simulink library "Surface_Mu_Axle3_LUT_Pos"  (R2026a)
settings: Solver=VariableStepAuto
undefined symbols (not defined in the file or in its folder): Scene
libraries: Tire_Utilities x6
Description:
  | Simscape Vehicle Templates Library
  | 
  | Copyright 2018-2024 The MathWorks, Inc.
settings Model: Creator=smiller  LastModifiedBy=smiller

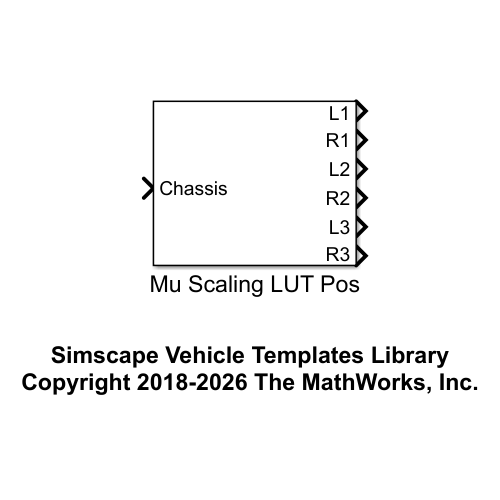
[thumbnail: Simulink's stored preview of the top-level diagram]
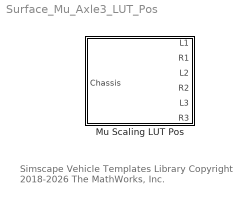
== system Surface_Mu_Axle3_LUT_Pos ==
  note: Simscape Vehicle Templates Library
      | Copyright 2018-2026 The MathWorks, Inc.
  Mu Scaling LUT Pos : Subsystem  VariantControl=Choice  mask(Scale Friction Coefficient by Position){xposL1=Scene.Mu_Scaling.x, yposL1=Scene.Mu_Scaling.y, ScaleTableL1=Scene.Mu_Scaling.scale, xposR1=Scene.Mu_Scaling.x, yposR1=Scene.Mu_Scaling.y, ScaleTableR1=Scene.Mu_Scaling.scale, xposL2=Scene.Mu_Scaling.x, yposL2=Scene.Mu_Scaling.y, ScaleTableL2=Scene.Mu_Scaling.scale, xposR2=Scene.Mu_Scaling.x, yposR2=Scene.Mu_Scaling.y, ScaleTableR2=Scene.Mu_Scaling.scale, xposL3=Scene.Mu_Scaling.x, yposL3=Scene.Mu_Scaling.y, ScaleTableL3=Scene.Mu_Scaling.scale, xposR3=Scene.Mu_Scaling.x, yposR3=Scene.Mu_Scaling.y, ScaleTableR3=Scene.Mu_Scaling.scale}
      mask help: Determines scaling factor for friction coefficient based on wheel x-y position.
      mask TypeOptions xposL1: LUT Scale L1/BreakpointsForDimension1
      mask TypeOptions yposL1: LUT Scale L1/BreakpointsForDimension2
      mask TypeOptions ScaleTableL1: LUT Scale L1/Table
      mask TypeOptions xposR1: LUT Scale R1/BreakpointsForDimension1
      mask TypeOptions yposR1: LUT Scale R1/BreakpointsForDimension2
      mask TypeOptions ScaleTableR1: LUT Scale R1/Table
      mask TypeOptions xposL2: LUT Scale L2/BreakpointsForDimension1
      mask TypeOptions yposL2: LUT Scale L2/BreakpointsForDimension2
      mask TypeOptions ScaleTableL2: LUT Scale L2/Table
      mask TypeOptions xposR2: LUT Scale R2/BreakpointsForDimension1
      mask TypeOptions yposR2: LUT Scale R2/BreakpointsForDimension2
      mask TypeOptions ScaleTableR2: LUT Scale R2/Table
      mask TypeOptions xposL3: LUT Scale L3/BreakpointsForDimension1
      mask TypeOptions yposL3: LUT Scale L3/BreakpointsForDimension2
      mask TypeOptions ScaleTableL3: LUT Scale L3/Table
      mask TypeOptions xposR3: LUT Scale R3/BreakpointsForDimension1
      mask TypeOptions yposR3: LUT Scale R3/BreakpointsForDimension2
      mask TypeOptions ScaleTableR3: LUT Scale R3/Table
      mask DialogControl text_whl Prompt: Wheel
      mask DialogControl text_xpos Prompt: X [1xm] (m)
      mask DialogControl text_ypos Prompt: Y [1xn] (m)
      mask DialogControl text_mu Prompt: Scale [mxn] (m)
      mask DialogControl text_L1 Prompt: L1
      mask DialogControl text_R1 Prompt: R1
      mask DialogControl text_L2 Prompt: L2
      mask DialogControl text_R2 Prompt: R2
      mask DialogControl text_L3 Prompt: L3
      mask DialogControl text_R3 Prompt: R3

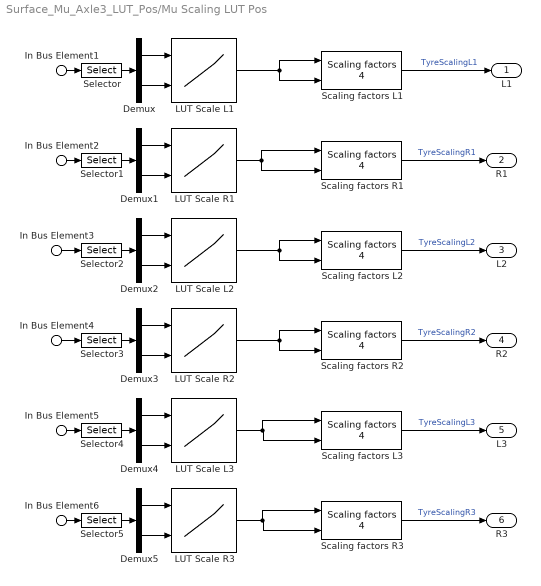
== system Surface_Mu_Axle3_LUT_Pos/Mu Scaling LUT Pos ==
  In Bus Element1 : Inport  PortName=Chassis  Element=WhlL1.xyz
  In Bus Element2 : Inport  PortName=Chassis  Element=WhlR1.xyz
  In Bus Element3 : Inport  PortName=Chassis  Element=WhlL2.xyz
  In Bus Element4 : Inport  PortName=Chassis  Element=WhlR2.xyz
  In Bus Element5 : Inport  PortName=Chassis  Element=WhlL3.xyz
  In Bus Element6 : Inport  PortName=Chassis  Element=WhlR3.xyz
  Demux{,1..5} (6 alike) : Demux  Outputs=2
  LUT Scale L1 : Lookup_n-D  BreakpointsForDimension1=xposL1  BreakpointsForDimension2=yposL1  Table=ScaleTableL1  InternalRulePriority=Speed  RndMeth=Simplest
      settings: InputPortMap=u0,u1
  LUT Scale L2 : Lookup_n-D  BreakpointsForDimension1=xposL2  BreakpointsForDimension2=yposL2  Table=ScaleTableL2  InternalRulePriority=Speed  RndMeth=Simplest
      settings: InputPortMap=u0,u1
  LUT Scale L3 : Lookup_n-D  BreakpointsForDimension1=xposL3  BreakpointsForDimension2=yposL3  Table=ScaleTableL3  InternalRulePriority=Speed  RndMeth=Simplest
      settings: InputPortMap=u0,u1
  LUT Scale R1 : Lookup_n-D  BreakpointsForDimension1=xposR1  BreakpointsForDimension2=yposR1  Table=ScaleTableR1  InternalRulePriority=Speed  RndMeth=Simplest
      settings: InputPortMap=u0,u1
  LUT Scale R2 : Lookup_n-D  BreakpointsForDimension1=xposR2  BreakpointsForDimension2=yposR2  Table=ScaleTableR2  InternalRulePriority=Speed  RndMeth=Simplest
      settings: InputPortMap=u0,u1
  LUT Scale R3 : Lookup_n-D  BreakpointsForDimension1=xposR3  BreakpointsForDimension2=yposR3  Table=ScaleTableR3  InternalRulePriority=Speed  RndMeth=Simplest
      settings: InputPortMap=u0,u1
  Scaling factors L1 : Tire_Utilities/Scaling factors 4  LKX=1  LKY=1  LKYC=1  LTR=1  LKZC=1
  Scaling factors L2 : Tire_Utilities/Scaling factors 4  LKX=1  LKY=1  LKYC=1  LTR=1  LKZC=1
  Scaling factors L3 : Tire_Utilities/Scaling factors 4  LKX=1  LKY=1  LKYC=1  LTR=1  LKZC=1
  Scaling factors R1 : Tire_Utilities/Scaling factors 4  LKX=1  LKY=1  LKYC=1  LTR=1  LKZC=1
  Scaling factors R2 : Tire_Utilities/Scaling factors 4  LKX=1  LKY=1  LKYC=1  LTR=1  LKZC=1
  Scaling factors R3 : Tire_Utilities/Scaling factors 4  LKX=1  LKY=1  LKYC=1  LTR=1  LKZC=1
  Selector{,1..5} (6 alike) : Selector  InputPortWidth=3  IndexOptions=Index vector (dialog)  Indices=[1 2]  OutputSizes=1
  L1 : Outport  VectorParamsAs1DForOutWhenUnconnected=off
  R1 : Outport  Port=2  VectorParamsAs1DForOutWhenUnconnected=off
  L2 : Outport  Port=3  VectorParamsAs1DForOutWhenUnconnected=off
  R2 : Outport  Port=4  VectorParamsAs1DForOutWhenUnconnected=off
  L3 : Outport  Port=5  VectorParamsAs1DForOutWhenUnconnected=off
  R3 : Outport  Port=6  VectorParamsAs1DForOutWhenUnconnected=off
  wires:
  In Bus Element1/1 -> Selector/1
  In Bus Element2/1 -> Selector1/1
  Selector/1 -> Demux/1
  Demux/2 -> LUT Scale L1/2
  Demux1/1 -> LUT Scale R1/1
  Demux1/2 -> LUT Scale R1/2
  Selector1/1 -> Demux1/1
  In Bus Element3/1 -> Selector2/1
  Demux2/1 -> LUT Scale L2/1
  Selector2/1 -> Demux2/1
  Demux2/2 -> LUT Scale L2/2
  In Bus Element4/1 -> Selector3/1
  Selector3/1 -> Demux3/1
  Demux3/1 -> LUT Scale R2/1
  Demux3/2 -> LUT Scale R2/2
  Demux/1 -> LUT Scale L1/1
  Scaling factors L2/1 -> L2/1  "TyreScalingL2"
  LUT Scale R3/1 -> Scaling factors R3/1, Scaling factors R3/2
  Scaling factors L3/1 -> L3/1  "TyreScalingL3"
  Scaling factors R2/1 -> R2/1  "TyreScalingR2"
  LUT Scale R2/1 -> Scaling factors R2/2, Scaling factors R2/1
  LUT Scale R1/1 -> Scaling factors R1/1, Scaling factors R1/2
  LUT Scale L2/1 -> Scaling factors L2/2, Scaling factors L2/1
  LUT Scale L1/1 -> Scaling factors L1/1, Scaling factors L1/2
  Scaling factors R1/1 -> R1/1  "TyreScalingR1"
  LUT Scale L3/1 -> Scaling factors L3/1, Scaling factors L3/2
  Scaling factors R3/1 -> R3/1  "TyreScalingR3"
  Scaling factors L1/1 -> L1/1  "TyreScalingL1"
  Demux5/2 -> LUT Scale R3/2
  Demux5/1 -> LUT Scale R3/1
  Selector5/1 -> Demux5/1
  Demux4/2 -> LUT Scale L3/2
  Selector4/1 -> Demux4/1
  Demux4/1 -> LUT Scale L3/1
  In Bus Element6/1 -> Selector5/1
  In Bus Element5/1 -> Selector4/1
